simulink model "pmc"  (Simulink 7.2)
settings: Solver=ode45  StartTime=0.0  StopTime=10.0  RelTol=1e-3
libraries: cdsFilt x9, cdsMuxMatrix x9, dac x2, cdsParameters x1
settings Model: Creator=rolf  LastModifiedBy=rolf  ExtModeAutoUpdateStatusClock=off
settings OptimizationCC: InitFltsAndDblsToZero=on
settings DebuggingCC: SaveWithParameterizedLinksMsg=none  SignalResolutionControl=TryResolveAllWithWarning
settings GRTTargetCC: TargetFcnLib=ansi_tfl_tmw.mat

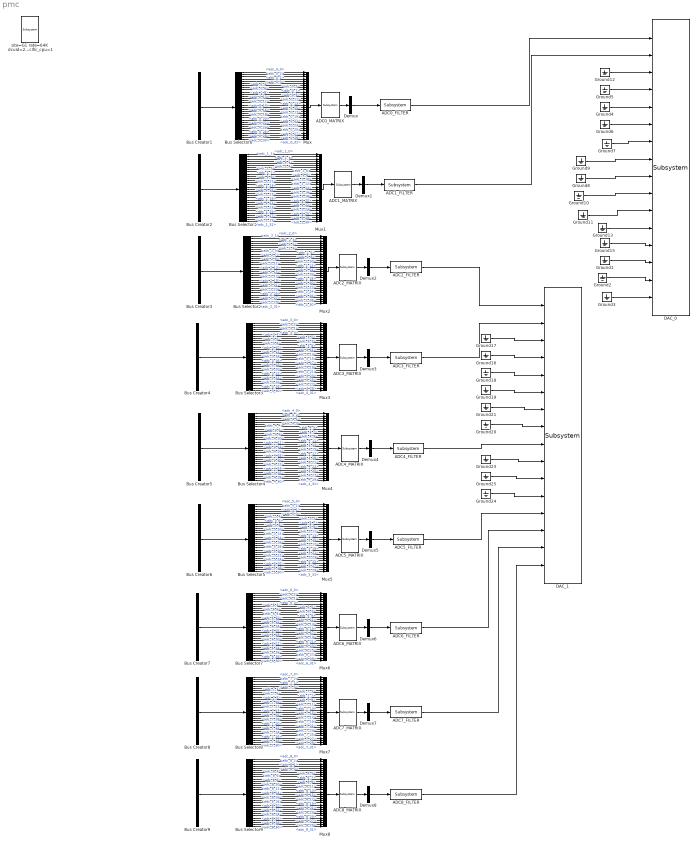
== system pmc ==
  ADC0_FILTER : cdsFilt/Subsystem  Tag=cdsFilt  Description=|  SystemSampleTime=-1
      | Purpose:                                                                                                                                                                                                                                  
      | Standard CDS IIR filter module.                                                                                                                                                                                                           
      |                                                                                                                                                                                                                                           
      | Operation:                                                                                                                                                                                                                                
      | Consists of 10 second order section IIR filters, plus a ramped gain stage. In FE code, also provides pre-defined test points and excitation channel inputs. The filter coefficients are defined in the LIGO system using the 'foton' tool.
      |                                                                                                                                                                                                                                           
      | Usage:                                                                                                                                                                                                                                    
      | Name the part with the desired filter module name.
      settings: AttributesFormatString=%<Tag>
  ADC0_MATRIX : cdsMuxMatrix/Subsystem  Tag=cdsMuxMatrix  Description=Any size matrix. Inputs and outputs must be connected using Mux and Demux parts.  SystemSampleTime=-1
      settings: AttributesFormatString=%<Tag>
  ADC1_FILTER : cdsFilt/Subsystem  Tag=cdsFilt  Description=|  SystemSampleTime=-1
      | Purpose:                                                                                                                                                                                                                                  
      | Standard CDS IIR filter module.                                                                                                                                                                                                           
      |                                                                                                                                                                                                                                           
      | Operation:                                                                                                                                                                                                                                
      | Consists of 10 second order section IIR filters, plus a ramped gain stage. In FE code, also provides pre-defined test points and excitation channel inputs. The filter coefficients are defined in the LIGO system using the 'foton' tool.
      |                                                                                                                                                                                                                                           
      | Usage:                                                                                                                                                                                                                                    
      | Name the part with the desired filter module name.
      settings: AttributesFormatString=%<Tag>
  ADC1_MATRIX : cdsMuxMatrix/Subsystem  Tag=cdsMuxMatrix  Description=Any size matrix. Inputs and outputs must be connected using Mux and Demux parts.  SystemSampleTime=-1
      settings: AttributesFormatString=%<Tag>
  ADC2_FILTER : cdsFilt/Subsystem  Tag=cdsFilt  Description=|  SystemSampleTime=-1
      | Purpose:                                                                                                                                                                                                                                  
      | Standard CDS IIR filter module.                                                                                                                                                                                                           
      |                                                                                                                                                                                                                                           
      | Operation:                                                                                                                                                                                                                                
      | Consists of 10 second order section IIR filters, plus a ramped gain stage. In FE code, also provides pre-defined test points and excitation channel inputs. The filter coefficients are defined in the LIGO system using the 'foton' tool.
      |                                                                                                                                                                                                                                           
      | Usage:                                                                                                                                                                                                                                    
      | Name the part with the desired filter module name.
      settings: AttributesFormatString=%<Tag>
  ADC2_MATRIX : cdsMuxMatrix/Subsystem  Tag=cdsMuxMatrix  Description=Any size matrix. Inputs and outputs must be connected using Mux and Demux parts.  SystemSampleTime=-1
      settings: AttributesFormatString=%<Tag>
  ADC3_FILTER : cdsFilt/Subsystem  Tag=cdsFilt  Description=|  SystemSampleTime=-1
      | Purpose:                                                                                                                                                                                                                                  
      | Standard CDS IIR filter module.                                                                                                                                                                                                           
      |                                                                                                                                                                                                                                           
      | Operation:                                                                                                                                                                                                                                
      | Consists of 10 second order section IIR filters, plus a ramped gain stage. In FE code, also provides pre-defined test points and excitation channel inputs. The filter coefficients are defined in the LIGO system using the 'foton' tool.
      |                                                                                                                                                                                                                                           
      | Usage:                                                                                                                                                                                                                                    
      | Name the part with the desired filter module name.
      settings: AttributesFormatString=%<Tag>
  ADC3_MATRIX : cdsMuxMatrix/Subsystem  Tag=cdsMuxMatrix  Description=Any size matrix. Inputs and outputs must be connected using Mux and Demux parts.  SystemSampleTime=-1
      settings: AttributesFormatString=%<Tag>
  ADC4_FILTER : cdsFilt/Subsystem  Tag=cdsFilt  Description=|  SystemSampleTime=-1
      | Purpose:                                                                                                                                                                                                                                  
      | Standard CDS IIR filter module.                                                                                                                                                                                                           
      |                                                                                                                                                                                                                                           
      | Operation:                                                                                                                                                                                                                                
      | Consists of 10 second order section IIR filters, plus a ramped gain stage. In FE code, also provides pre-defined test points and excitation channel inputs. The filter coefficients are defined in the LIGO system using the 'foton' tool.
      |                                                                                                                                                                                                                                           
      | Usage:                                                                                                                                                                                                                                    
      | Name the part with the desired filter module name.
      settings: AttributesFormatString=%<Tag>
  ADC4_MATRIX : cdsMuxMatrix/Subsystem  Tag=cdsMuxMatrix  Description=Any size matrix. Inputs and outputs must be connected using Mux and Demux parts.  SystemSampleTime=-1
      settings: AttributesFormatString=%<Tag>
  ADC5_FILTER : cdsFilt/Subsystem  Tag=cdsFilt  Description=|  SystemSampleTime=-1
      | Purpose:                                                                                                                                                                                                                                  
      | Standard CDS IIR filter module.                                                                                                                                                                                                           
      |                                                                                                                                                                                                                                           
      | Operation:                                                                                                                                                                                                                                
      | Consists of 10 second order section IIR filters, plus a ramped gain stage. In FE code, also provides pre-defined test points and excitation channel inputs. The filter coefficients are defined in the LIGO system using the 'foton' tool.
      |                                                                                                                                                                                                                                           
      | Usage:                                                                                                                                                                                                                                    
      | Name the part with the desired filter module name.
      settings: AttributesFormatString=%<Tag>
  ADC5_MATRIX : cdsMuxMatrix/Subsystem  Tag=cdsMuxMatrix  Description=Any size matrix. Inputs and outputs must be connected using Mux and Demux parts.  SystemSampleTime=-1
      settings: AttributesFormatString=%<Tag>
  ADC6_FILTER : cdsFilt/Subsystem  Tag=cdsFilt  Description=|  SystemSampleTime=-1
      | Purpose:                                                                                                                                                                                                                                  
      | Standard CDS IIR filter module.                                                                                                                                                                                                           
      |                                                                                                                                                                                                                                           
      | Operation:                                                                                                                                                                                                                                
      | Consists of 10 second order section IIR filters, plus a ramped gain stage. In FE code, also provides pre-defined test points and excitation channel inputs. The filter coefficients are defined in the LIGO system using the 'foton' tool.
      |                                                                                                                                                                                                                                           
      | Usage:                                                                                                                                                                                                                                    
      | Name the part with the desired filter module name.
      settings: AttributesFormatString=%<Tag>
  ADC6_MATRIX : cdsMuxMatrix/Subsystem  Tag=cdsMuxMatrix  Description=Any size matrix. Inputs and outputs must be connected using Mux and Demux parts.  SystemSampleTime=-1
      settings: AttributesFormatString=%<Tag>
  ADC7_FILTER : cdsFilt/Subsystem  Tag=cdsFilt  Description=|  SystemSampleTime=-1
      | Purpose:                                                                                                                                                                                                                                  
      | Standard CDS IIR filter module.                                                                                                                                                                                                           
      |                                                                                                                                                                                                                                           
      | Operation:                                                                                                                                                                                                                                
      | Consists of 10 second order section IIR filters, plus a ramped gain stage. In FE code, also provides pre-defined test points and excitation channel inputs. The filter coefficients are defined in the LIGO system using the 'foton' tool.
      |                                                                                                                                                                                                                                           
      | Usage:                                                                                                                                                                                                                                    
      | Name the part with the desired filter module name.
      settings: AttributesFormatString=%<Tag>
  ADC7_MATRIX : cdsMuxMatrix/Subsystem  Tag=cdsMuxMatrix  Description=Any size matrix. Inputs and outputs must be connected using Mux and Demux parts.  SystemSampleTime=-1
      settings: AttributesFormatString=%<Tag>
  ADC8_FILTER : cdsFilt/Subsystem  Tag=cdsFilt  Description=|  SystemSampleTime=-1
      | Purpose:                                                                                                                                                                                                                                  
      | Standard CDS IIR filter module.                                                                                                                                                                                                           
      |                                                                                                                                                                                                                                           
      | Operation:                                                                                                                                                                                                                                
      | Consists of 10 second order section IIR filters, plus a ramped gain stage. In FE code, also provides pre-defined test points and excitation channel inputs. The filter coefficients are defined in the LIGO system using the 'foton' tool.
      |                                                                                                                                                                                                                                           
      | Usage:                                                                                                                                                                                                                                    
      | Name the part with the desired filter module name.
      settings: AttributesFormatString=%<Tag>
  ADC8_MATRIX : cdsMuxMatrix/Subsystem  Tag=cdsMuxMatrix  Description=Any size matrix. Inputs and outputs must be connected using Mux and Demux parts.  SystemSampleTime=-1
      settings: AttributesFormatString=%<Tag>
  Bus Creator1 : BusCreator  Tag=adc_0  Description=|  Inputs='adc_0_0','adc_0_1','adc_0_2','adc_0_3','adc_0_4','adc_0_5','adc_0_6','adc_0_7','adc_0_8','adc_0_9','adc_0_10','adc_0_11','adc_0_12','adc_0_13','adc_0_14','adc_0_15','adc_0_16','adc_0_17','adc_0_18','adc_0_19','adc_0_20','adc_0_21','adc_0_22','adc_0_23','adc_0_24','adc_0_25','adc_0_26','adc_0_27','adc_0_28','adc_0_29','adc_0_30','adc_0_31'
      | ADC0      
      | card_num=0
      settings: AttributesFormatString=%<Description>
  Bus Creator2 : BusCreator  Description=|  Inputs='adc_1_0','adc_1_1','adc_1_2','adc_1_3','adc_1_4','adc_1_5','adc_1_6','adc_1_7','adc_1_8','adc_1_9','adc_1_10','adc_1_11','adc_1_12','adc_1_13','adc_1_14','adc_1_15','adc_1_16','adc_1_17','adc_1_18','adc_1_19','adc_1_20','adc_1_21','adc_1_22','adc_1_23','adc_1_24','adc_1_25','adc_1_26','adc_1_27','adc_1_28','adc_1_29','adc_1_30','adc_1_31'
      | ADC1      
      | card_num=1
      settings: AttributesFormatString=%<Description>
  Bus Creator3 : BusCreator  Description=|  Inputs='adc_2_0','adc_2_1','adc_2_2','adc_2_3','adc_2_4','adc_2_5','adc_2_6','adc_2_7','adc_2_8','adc_2_9','adc_2_10','adc_2_11','adc_2_12','adc_2_13','adc_2_14','adc_2_15','adc_2_16','adc_2_17','adc_2_18','adc_2_19','adc_2_20','adc_2_21','adc_2_22','adc_2_23','adc_2_24','adc_2_25','adc_2_26','adc_2_27','adc_2_28','adc_2_29','adc_2_30','adc_2_31'
      | ADC2      
      | card_num=2
      settings: AttributesFormatString=%<Description>
  Bus Creator4 : BusCreator  Description=|  Inputs='adc_3_0','adc_3_1','adc_3_2','adc_3_3','adc_3_4','adc_3_5','adc_3_6','adc_3_7','adc_3_8','adc_3_9','adc_3_10','adc_3_11','adc_3_12','adc_3_13','adc_3_14','adc_3_15','adc_3_16','adc_3_17','adc_3_18','adc_3_19','adc_3_20','adc_3_21','adc_3_22','adc_3_23','adc_3_24','adc_3_25','adc_3_26','adc_3_27','adc_3_28','adc_3_29','adc_3_30','adc_3_31'
      | ADC3      
      | card_num=3
      settings: AttributesFormatString=%<Description>
  Bus Creator5 : BusCreator  Description=|  Inputs='adc_4_0','adc_4_1','adc_4_2','adc_4_3','adc_4_4','adc_4_5','adc_4_6','adc_4_7','adc_4_8','adc_4_9','adc_4_10','adc_4_11','adc_4_12','adc_4_13','adc_4_14','adc_4_15','adc_4_16','adc_4_17','adc_4_18','adc_4_19','adc_4_20','adc_4_21','adc_4_22','adc_4_23','adc_4_24','adc_4_25','adc_4_26','adc_4_27','adc_4_28','adc_4_29','adc_4_30','adc_4_31'
      | ADC4      
      | card_num=4
      settings: AttributesFormatString=%<Description>
  Bus Creator6 : BusCreator  Description=|  Inputs='adc_5_0','adc_5_1','adc_5_2','adc_5_3','adc_5_4','adc_5_5','adc_5_6','adc_5_7','adc_5_8','adc_5_9','adc_5_10','adc_5_11','adc_5_12','adc_5_13','adc_5_14','adc_5_15','adc_5_16','adc_5_17','adc_5_18','adc_5_19','adc_5_20','adc_5_21','adc_5_22','adc_5_23','adc_5_24','adc_5_25','adc_5_26','adc_5_27','adc_5_28','adc_5_29','adc_5_30','adc_5_31'
      | ADC5      
      | card_num=5
      settings: AttributesFormatString=%<Description>
  Bus Creator7 : BusCreator  Description=|  Inputs='adc_6_0','adc_6_1','adc_6_2','adc_6_3','adc_6_4','adc_6_5','adc_6_6','adc_6_7','adc_6_8','adc_6_9','adc_6_10','adc_6_11','adc_6_12','adc_6_13','adc_6_14','adc_6_15','adc_6_16','adc_6_17','adc_6_18','adc_6_19','adc_6_20','adc_6_21','adc_6_22','adc_6_23','adc_6_24','adc_6_25','adc_6_26','adc_6_27','adc_6_28','adc_6_29','adc_6_30','adc_6_31'
      | ADC6      
      | card_num=6
      settings: AttributesFormatString=%<Description>
  Bus Creator8 : BusCreator  Description=|  Inputs='adc_7_0','adc_7_1','adc_7_2','adc_7_3','adc_7_4','adc_7_5','adc_7_6','adc_7_7','adc_7_8','adc_7_9','adc_7_10','adc_7_11','adc_7_12','adc_7_13','adc_7_14','adc_7_15','adc_7_16','adc_7_17','adc_7_18','adc_7_19','adc_7_20','adc_7_21','adc_7_22','adc_7_23','adc_7_24','adc_7_25','adc_7_26','adc_7_27','adc_7_28','adc_7_29','adc_7_30','adc_7_31'
      | ADC7      
      | card_num=7
      settings: AttributesFormatString=%<Description>
  Bus Creator9 : BusCreator  Description=|  Inputs='adc_8_0','adc_8_1','adc_8_2','adc_8_3','adc_8_4','adc_8_5','adc_8_6','adc_8_7','adc_8_8','adc_8_9','adc_8_10','adc_8_11','adc_8_12','adc_8_13','adc_8_14','adc_8_15','adc_8_16','adc_8_17','adc_8_18','adc_8_19','adc_8_20','adc_8_21','adc_8_22','adc_8_23','adc_8_24','adc_8_25','adc_8_26','adc_8_27','adc_8_28','adc_8_29','adc_8_30','adc_8_31'
      | ADC8      
      | card_num=8
      settings: AttributesFormatString=%<Description>
  Bus Selector1 : BusSelector  Description=ADC Selector  OutputSignals=adc_1_0,adc_1_1,adc_1_2,adc_1_3,adc_1_4,adc_1_5,adc_1_6,adc_1_7,adc_1_8,adc_1_9,adc_1_10,adc_1_11,adc_1_12,adc_1_13,adc_1_14,adc_1_15,adc_1_16,adc_1_17,adc_1_18,adc_1_19,adc_1_20,adc_1_21,adc_1_22,adc_1_23,adc_1_24,adc_1_25,adc_1_26,adc_1_27,adc_1_28,adc_1_29,adc_1_30,adc_1_31
      settings: AttributesFormatString=%<Description>
  Bus Selector2 : BusSelector  Description=ADC Selector  OutputSignals=adc_2_0,adc_2_1,adc_2_2,adc_2_3,adc_2_4,adc_2_5,adc_2_6,adc_2_7,adc_2_8,adc_2_9,adc_2_10,adc_2_11,adc_2_12,adc_2_13,adc_2_14,adc_2_15,adc_2_16,adc_2_17,adc_2_18,adc_2_19,adc_2_20,adc_2_21,adc_2_22,adc_2_23,adc_2_24,adc_2_25,adc_2_26,adc_2_27,adc_2_28,adc_2_29,adc_2_30,adc_2_31
      settings: AttributesFormatString=%<Description>
  Bus Selector3 : BusSelector  Description=ADC Selector  OutputSignals=adc_3_0,adc_3_1,adc_3_2,adc_3_3,adc_3_4,adc_3_5,adc_3_6,adc_3_7,adc_3_8,adc_3_9,adc_3_10,adc_3_11,adc_3_12,adc_3_13,adc_3_14,adc_3_15,adc_3_16,adc_3_17,adc_3_18,adc_3_19,adc_3_20,adc_3_21,adc_3_22,adc_3_23,adc_3_24,adc_3_25,adc_3_26,adc_3_27,adc_3_28,adc_3_29,adc_3_30,adc_3_31
      settings: AttributesFormatString=%<Description>
  Bus Selector4 : BusSelector  Description=ADC Selector  OutputSignals=adc_4_0,adc_4_1,adc_4_2,adc_4_3,adc_4_4,adc_4_5,adc_4_6,adc_4_7,adc_4_8,adc_4_9,adc_4_10,adc_4_11,adc_4_12,adc_4_13,adc_4_14,adc_4_15,adc_4_16,adc_4_17,adc_4_18,adc_4_19,adc_4_20,adc_4_21,adc_4_22,adc_4_23,adc_4_24,adc_4_25,adc_4_26,adc_4_27,adc_4_28,adc_4_29,adc_4_30,adc_4_31
      settings: AttributesFormatString=%<Description>
  Bus Selector5 : BusSelector  Description=ADC Selector  OutputSignals=adc_5_0,adc_5_1,adc_5_2,adc_5_3,adc_5_4,adc_5_5,adc_5_6,adc_5_7,adc_5_8,adc_5_9,adc_5_10,adc_5_11,adc_5_12,adc_5_13,adc_5_14,adc_5_15,adc_5_16,adc_5_17,adc_5_18,adc_5_19,adc_5_20,adc_5_21,adc_5_22,adc_5_23,adc_5_24,adc_5_25,adc_5_26,adc_5_27,adc_5_28,adc_5_29,adc_5_30,adc_5_31
      settings: AttributesFormatString=%<Description>
  Bus Selector6 : BusSelector  Description=ADC Selector  OutputSignals=adc_0_0,adc_0_1,adc_0_2,adc_0_3,adc_0_4,adc_0_5,adc_0_6,adc_0_7,adc_0_8,adc_0_9,adc_0_10,adc_0_11,adc_0_12,adc_0_13,adc_0_14,adc_0_15,adc_0_16,adc_0_17,adc_0_18,adc_0_19,adc_0_20,adc_0_21,adc_0_22,adc_0_23,adc_0_24,adc_0_25,adc_0_26,adc_0_27,adc_0_28,adc_0_29,adc_0_30,adc_0_31
      settings: AttributesFormatString=%<Description>
  Bus Selector7 : BusSelector  Description=ADC Selector  OutputSignals=adc_6_0,adc_6_1,adc_6_2,adc_6_3,adc_6_4,adc_6_5,adc_6_6,adc_6_7,adc_6_8,adc_6_9,adc_6_10,adc_6_11,adc_6_12,adc_6_13,adc_6_14,adc_6_15,adc_6_16,adc_6_17,adc_6_18,adc_6_19,adc_6_20,adc_6_21,adc_6_22,adc_6_23,adc_6_24,adc_6_25,adc_6_26,adc_6_27,adc_6_28,adc_6_29,adc_6_30,adc_6_31
      settings: AttributesFormatString=%<Description>
  Bus Selector8 : BusSelector  Description=ADC Selector  OutputSignals=adc_7_0,adc_7_1,adc_7_2,adc_7_3,adc_7_4,adc_7_5,adc_7_6,adc_7_7,adc_7_8,adc_7_9,adc_7_10,adc_7_11,adc_7_12,adc_7_13,adc_7_14,adc_7_15,adc_7_16,adc_7_17,adc_7_18,adc_7_19,adc_7_20,adc_7_21,adc_7_22,adc_7_23,adc_7_24,adc_7_25,adc_7_26,adc_7_27,adc_7_28,adc_7_29,adc_7_30,adc_7_31
      settings: AttributesFormatString=%<Description>
  Bus Selector9 : BusSelector  Description=ADC Selector  OutputSignals=adc_8_0,adc_8_1,adc_8_2,adc_8_3,adc_8_4,adc_8_5,adc_8_6,adc_8_7,adc_8_8,adc_8_9,adc_8_10,adc_8_11,adc_8_12,adc_8_13,adc_8_14,adc_8_15,adc_8_16,adc_8_17,adc_8_18,adc_8_19,adc_8_20,adc_8_21,adc_8_22,adc_8_23,adc_8_24,adc_8_25,adc_8_26,adc_8_27,adc_8_28,adc_8_29,adc_8_30,adc_8_31
      settings: AttributesFormatString=%<Description>
  DAC_0 : dac/Subsystem  Description=card_num=0  SystemSampleTime=-1
  DAC_1 : dac/Subsystem  Description=card_num=1  SystemSampleTime=-1
  Demux{,1..8} (9 alike) : Demux  Outputs=1
  Ground{1..13,15..21,23..25} (23 alike) : Ground
  Mux{,1..8} (9 alike) : Mux  Inputs=32
  site=G1 rate=64K dcuid=20 shmem_daq=1 gds_node_id=4 specific_cpu=1 : cdsParameters/Subsystem  Tag=cdsParameters  SystemSampleTime=-1
      settings: AttributesFormatString=%<Tag>
  wires:
  Ground15/1 -> DAC_0/13
  Ground1/1 -> DAC_0/14
  Ground2/1 -> DAC_0/15
  Ground3/1 -> DAC_0/16
  Bus Creator1/1 -> Bus Selector6/1
  Bus Creator2/1 -> Bus Selector1/1
  Bus Creator3/1 -> Bus Selector2/1
  Mux/1 -> ADC0_MATRIX/1
  ADC0_MATRIX/1 -> Demux/1
  Bus Selector6/1 -> Mux/1  "<adc_0_0>"
  Bus Selector6/2 -> Mux/2  "<adc_0_1>"
  Bus Selector6/3 -> Mux/3  "<adc_0_2>"
  Bus Selector6/4 -> Mux/4  "<adc_0_3>"
  Bus Selector6/5 -> Mux/5  "<adc_0_4>"
  Bus Selector6/6 -> Mux/6  "<adc_0_5>"
  Bus Selector6/7 -> Mux/7  "<adc_0_6>"
  Bus Selector6/8 -> Mux/8  "<adc_0_7>"
  Bus Selector6/9 -> Mux/9  "<adc_0_8>"
  Bus Selector6/10 -> Mux/10  "<adc_0_9>"
  Bus Selector6/11 -> Mux/11  "<adc_0_10>"
  Bus Selector6/12 -> Mux/12  "<adc_0_11>"
  Bus Selector6/13 -> Mux/13  "<adc_0_12>"
  Bus Selector6/14 -> Mux/14  "<adc_0_13>"
  Bus Selector6/15 -> Mux/15  "<adc_0_14>"
  Bus Selector6/16 -> Mux/16  "<adc_0_15>"
  Bus Selector6/17 -> Mux/17  "<adc_0_16>"
  Bus Selector6/18 -> Mux/18  "<adc_0_17>"
  Bus Selector6/19 -> Mux/19  "<adc_0_18>"
  Bus Selector6/20 -> Mux/20  "<adc_0_19>"
  Bus Selector6/21 -> Mux/21  "<adc_0_20>"
  Bus Selector6/22 -> Mux/22  "<adc_0_21>"
  Bus Selector6/23 -> Mux/23  "<adc_0_22>"
  Bus Selector6/24 -> Mux/24  "<adc_0_23>"
  Bus Selector6/25 -> Mux/25  "<adc_0_24>"
  Bus Selector6/26 -> Mux/26  "<adc_0_25>"
  Bus Selector6/27 -> Mux/27  "<adc_0_26>"
  Bus Selector6/28 -> Mux/28  "<adc_0_27>"
  Bus Selector6/29 -> Mux/29  "<adc_0_28>"
  Bus Selector6/30 -> Mux/30  "<adc_0_29>"
  Bus Selector6/31 -> Mux/31  "<adc_0_30>"
  Bus Selector6/32 -> Mux/32  "<adc_0_31>"
  Demux/1 -> ADC0_FILTER/1
  Mux1/1 -> ADC1_MATRIX/1
  ADC1_MATRIX/1 -> Demux1/1
  Bus Selector1/1 -> Mux1/1  "<adc_1_0>"
  Bus Selector1/2 -> Mux1/2  "<adc_1_1>"
  Bus Selector1/3 -> Mux1/3  "<adc_1_2>"
  Bus Selector1/4 -> Mux1/4  "<adc_1_3>"
  Bus Selector1/5 -> Mux1/5  "<adc_1_4>"
  Bus Selector1/6 -> Mux1/6  "<adc_1_5>"
  Bus Selector1/7 -> Mux1/7  "<adc_1_6>"
  Bus Selector1/8 -> Mux1/8  "<adc_1_7>"
  Bus Selector1/9 -> Mux1/9  "<adc_1_8>"
  Bus Selector1/10 -> Mux1/10  "<adc_1_9>"
  Bus Selector1/11 -> Mux1/11  "<adc_1_10>"
  Bus Selector1/12 -> Mux1/12  "<adc_1_11>"
  Bus Selector1/13 -> Mux1/13  "<adc_1_12>"
  Bus Selector1/14 -> Mux1/14  "<adc_1_13>"
  Bus Selector1/15 -> Mux1/15  "<adc_1_14>"
  Bus Selector1/16 -> Mux1/16  "<adc_1_15>"
  Bus Selector1/17 -> Mux1/17  "<adc_1_16>"
  Bus Selector1/18 -> Mux1/18  "<adc_1_17>"
  Bus Selector1/19 -> Mux1/19  "<adc_1_18>"
  Bus Selector1/20 -> Mux1/20  "<adc_1_19>"
  Bus Selector1/21 -> Mux1/21  "<adc_1_20>"
  Bus Selector1/22 -> Mux1/22  "<adc_1_21>"
  Bus Selector1/23 -> Mux1/23  "<adc_1_22>"
  Bus Selector1/24 -> Mux1/24  "<adc_1_23>"
  Bus Selector1/25 -> Mux1/25  "<adc_1_24>"
  Bus Selector1/26 -> Mux1/26  "<adc_1_25>"
  Bus Selector1/27 -> Mux1/27  "<adc_1_26>"
  Bus Selector1/28 -> Mux1/28  "<adc_1_27>"
  Bus Selector1/29 -> Mux1/29  "<adc_1_28>"
  Bus Selector1/30 -> Mux1/30  "<adc_1_29>"
  Bus Selector1/31 -> Mux1/31  "<adc_1_30>"
  Bus Selector1/32 -> Mux1/32  "<adc_1_31>"
  Mux2/1 -> ADC2_MATRIX/1
  ADC2_MATRIX/1 -> Demux2/1
  Bus Selector2/1 -> Mux2/1  "<adc_2_0>"
  Bus Selector2/2 -> Mux2/2  "<adc_2_1>"
  Bus Selector2/3 -> Mux2/3  "<adc_2_2>"
  Bus Selector2/4 -> Mux2/4  "<adc_2_3>"
  Bus Selector2/5 -> Mux2/5  "<adc_2_4>"
  Bus Selector2/6 -> Mux2/6  "<adc_2_5>"
  Bus Selector2/7 -> Mux2/7  "<adc_2_6>"
  Bus Selector2/8 -> Mux2/8  "<adc_2_7>"
  Bus Selector2/9 -> Mux2/9  "<adc_2_8>"
  Bus Selector2/10 -> Mux2/10  "<adc_2_9>"
  Bus Selector2/11 -> Mux2/11  "<adc_2_10>"
  Bus Selector2/12 -> Mux2/12  "<adc_2_11>"
  Bus Selector2/13 -> Mux2/13  "<adc_2_12>"
  Bus Selector2/14 -> Mux2/14  "<adc_2_13>"
  Bus Selector2/15 -> Mux2/15  "<adc_2_14>"
  Bus Selector2/16 -> Mux2/16  "<adc_2_15>"
  Bus Selector2/17 -> Mux2/17  "<adc_2_16>"
  Bus Selector2/18 -> Mux2/18  "<adc_2_17>"
  Bus Selector2/19 -> Mux2/19  "<adc_2_18>"
  Bus Selector2/20 -> Mux2/20  "<adc_2_19>"
  Bus Selector2/21 -> Mux2/21  "<adc_2_20>"
  Bus Selector2/22 -> Mux2/22  "<adc_2_21>"
  Bus Selector2/23 -> Mux2/23  "<adc_2_22>"
  Bus Selector2/24 -> Mux2/24  "<adc_2_23>"
  Bus Selector2/25 -> Mux2/25  "<adc_2_24>"
  Bus Selector2/26 -> Mux2/26  "<adc_2_25>"
  Bus Selector2/27 -> Mux2/27  "<adc_2_26>"
  Bus Selector2/28 -> Mux2/28  "<adc_2_27>"
  Bus Selector2/29 -> Mux2/29  "<adc_2_28>"
  Bus Selector2/30 -> Mux2/30  "<adc_2_29>"
  Bus Selector2/31 -> Mux2/31  "<adc_2_30>"
  Bus Selector2/32 -> Mux2/32  "<adc_2_31>"
  Demux2/1 -> ADC2_FILTER/1
  Demux1/1 -> ADC1_FILTER/1
  ADC0_FILTER/1 -> DAC_0/1
  ADC1_FILTER/1 -> DAC_0/2
  Ground5/1 -> DAC_0/4
  Ground4/1 -> DAC_0/5
  Ground6/1 -> DAC_0/6
  Ground7/1 -> DAC_0/7
  Ground9/1 -> DAC_0/8
  Ground8/1 -> DAC_0/9
  Ground10/1 -> DAC_0/10
  Ground11/1 -> DAC_0/11
  Ground13/1 -> DAC_0/12
  ADC2_FILTER/1 -> DAC_1/1
  Ground12/1 -> DAC_0/3
  Ground17/1 -> DAC_1/3
  Ground16/1 -> DAC_1/4
  Ground18/1 -> DAC_1/5
  Ground19/1 -> DAC_1/6
  Ground21/1 -> DAC_1/7
  Ground20/1 -> DAC_1/8
  Ground23/1 -> DAC_1/10
  Ground25/1 -> DAC_1/11
  Ground24/1 -> DAC_1/12
  Bus Creator4/1 -> Bus Selector3/1
  Mux3/1 -> ADC3_MATRIX/1
  ADC3_MATRIX/1 -> Demux3/1
  Demux3/1 -> ADC3_FILTER/1
  Bus Selector3/1 -> Mux3/1  "<adc_3_0>"
  Bus Selector3/2 -> Mux3/2  "<adc_3_1>"
  Bus Selector3/3 -> Mux3/3  "<adc_3_2>"
  Bus Selector3/4 -> Mux3/4  "<adc_3_3>"
  Bus Selector3/5 -> Mux3/5  "<adc_3_4>"
  Bus Selector3/6 -> Mux3/6  "<adc_3_5>"
  Bus Selector3/7 -> Mux3/7  "<adc_3_6>"
  Bus Selector3/8 -> Mux3/8  "<adc_3_7>"
  Bus Selector3/9 -> Mux3/9  "<adc_3_8>"
  Bus Selector3/10 -> Mux3/10  "<adc_3_9>"
  Bus Selector3/11 -> Mux3/11  "<adc_3_10>"
  Bus Selector3/12 -> Mux3/12  "<adc_3_11>"
  Bus Selector3/13 -> Mux3/13  "<adc_3_12>"
  Bus Selector3/14 -> Mux3/14  "<adc_3_13>"
  Bus Selector3/15 -> Mux3/15  "<adc_3_14>"
  Bus Selector3/16 -> Mux3/16  "<adc_3_15>"
  Bus Selector3/17 -> Mux3/17  "<adc_3_16>"
  Bus Selector3/18 -> Mux3/18  "<adc_3_17>"
  Bus Selector3/19 -> Mux3/19  "<adc_3_18>"
  Bus Selector3/20 -> Mux3/20  "<adc_3_19>"
  Bus Selector3/21 -> Mux3/21  "<adc_3_20>"
  Bus Selector3/22 -> Mux3/22  "<adc_3_21>"
  Bus Selector3/23 -> Mux3/23  "<adc_3_22>"
  Bus Selector3/24 -> Mux3/24  "<adc_3_23>"
  Bus Selector3/25 -> Mux3/25  "<adc_3_24>"
  Bus Selector3/26 -> Mux3/26  "<adc_3_25>"
  Bus Selector3/27 -> Mux3/27  "<adc_3_26>"
  Bus Selector3/28 -> Mux3/28  "<adc_3_27>"
  Bus Selector3/29 -> Mux3/29  "<adc_3_28>"
  Bus Selector3/30 -> Mux3/30  "<adc_3_29>"
  Bus Selector3/31 -> Mux3/31  "<adc_3_30>"
  Bus Selector3/32 -> Mux3/32  "<adc_3_31>"
  ADC3_FILTER/1 -> DAC_1/2
  Bus Creator5/1 -> Bus Selector4/1
  Mux4/1 -> ADC4_MATRIX/1
  ADC4_MATRIX/1 -> Demux4/1
  Demux4/1 -> ADC4_FILTER/1
  Bus Selector4/1 -> Mux4/1  "<adc_4_0>"
  Bus Selector4/2 -> Mux4/2  "<adc_4_1>"
  Bus Selector4/3 -> Mux4/3  "<adc_4_2>"
  Bus Selector4/4 -> Mux4/4  "<adc_4_3>"
  Bus Selector4/5 -> Mux4/5  "<adc_4_4>"
  Bus Selector4/6 -> Mux4/6  "<adc_4_5>"
  Bus Selector4/7 -> Mux4/7  "<adc_4_6>"
  Bus Selector4/8 -> Mux4/8  "<adc_4_7>"
  Bus Selector4/9 -> Mux4/9  "<adc_4_8>"
  Bus Selector4/10 -> Mux4/10  "<adc_4_9>"
  Bus Selector4/11 -> Mux4/11  "<adc_4_10>"
  Bus Selector4/12 -> Mux4/12  "<adc_4_11>"
  Bus Selector4/13 -> Mux4/13  "<adc_4_12>"
  Bus Selector4/14 -> Mux4/14  "<adc_4_13>"
  Bus Selector4/15 -> Mux4/15  "<adc_4_14>"
  Bus Selector4/16 -> Mux4/16  "<adc_4_15>"
  Bus Selector4/17 -> Mux4/17  "<adc_4_16>"
  Bus Selector4/18 -> Mux4/18  "<adc_4_17>"
  Bus Selector4/19 -> Mux4/19  "<adc_4_18>"
  Bus Selector4/20 -> Mux4/20  "<adc_4_19>"
  Bus Selector4/21 -> Mux4/21  "<adc_4_20>"
  Bus Selector4/22 -> Mux4/22  "<adc_4_21>"
  Bus Selector4/23 -> Mux4/23  "<adc_4_22>"
  Bus Selector4/24 -> Mux4/24  "<adc_4_23>"
  Bus Selector4/25 -> Mux4/25  "<adc_4_24>"
  Bus Selector4/26 -> Mux4/26  "<adc_4_25>"
  Bus Selector4/27 -> Mux4/27  "<adc_4_26>"
  Bus Selector4/28 -> Mux4/28  "<adc_4_27>"
  Bus Selector4/29 -> Mux4/29  "<adc_4_28>"
  Bus Selector4/30 -> Mux4/30  "<adc_4_29>"
  Bus Selector4/31 -> Mux4/31  "<adc_4_30>"
  Bus Selector4/32 -> Mux4/32  "<adc_4_31>"
  ADC4_FILTER/1 -> DAC_1/9
  Bus Creator6/1 -> Bus Selector5/1
  Mux5/1 -> ADC5_MATRIX/1
  ADC5_MATRIX/1 -> Demux5/1
  Demux5/1 -> ADC5_FILTER/1
  Bus Selector5/1 -> Mux5/1  "<adc_5_0>"
  Bus Selector5/2 -> Mux5/2  "<adc_5_1>"
  Bus Selector5/3 -> Mux5/3  "<adc_5_2>"
  Bus Selector5/4 -> Mux5/4  "<adc_5_3>"
  Bus Selector5/5 -> Mux5/5  "<adc_5_4>"
  Bus Selector5/6 -> Mux5/6  "<adc_5_5>"
  Bus Selector5/7 -> Mux5/7  "<adc_5_6>"
  Bus Selector5/8 -> Mux5/8  "<adc_5_7>"
  Bus Selector5/9 -> Mux5/9  "<adc_5_8>"
  Bus Selector5/10 -> Mux5/10  "<adc_5_9>"
  Bus Selector5/11 -> Mux5/11  "<adc_5_10>"
  Bus Selector5/12 -> Mux5/12  "<adc_5_11>"
  Bus Selector5/13 -> Mux5/13  "<adc_5_12>"
  Bus Selector5/14 -> Mux5/14  "<adc_5_13>"
  Bus Selector5/15 -> Mux5/15  "<adc_5_14>"
  Bus Selector5/16 -> Mux5/16  "<adc_5_15>"
  Bus Selector5/17 -> Mux5/17  "<adc_5_16>"
  Bus Selector5/18 -> Mux5/18  "<adc_5_17>"
  Bus Selector5/19 -> Mux5/19  "<adc_5_18>"
  Bus Selector5/20 -> Mux5/20  "<adc_5_19>"
  Bus Selector5/21 -> Mux5/21  "<adc_5_20>"
  Bus Selector5/22 -> Mux5/22  "<adc_5_21>"
  Bus Selector5/23 -> Mux5/23  "<adc_5_22>"
  Bus Selector5/24 -> Mux5/24  "<adc_5_23>"
  Bus Selector5/25 -> Mux5/25  "<adc_5_24>"
  Bus Selector5/26 -> Mux5/26  "<adc_5_25>"
  Bus Selector5/27 -> Mux5/27  "<adc_5_26>"
  Bus Selector5/28 -> Mux5/28  "<adc_5_27>"
  Bus Selector5/29 -> Mux5/29  "<adc_5_28>"
  Bus Selector5/30 -> Mux5/30  "<adc_5_29>"
  Bus Selector5/31 -> Mux5/31  "<adc_5_30>"
  Bus Selector5/32 -> Mux5/32  "<adc_5_31>"
  ADC5_FILTER/1 -> DAC_1/13
  Bus Creator7/1 -> Bus Selector7/1
  Mux6/1 -> ADC6_MATRIX/1
  ADC6_MATRIX/1 -> Demux6/1
  Demux6/1 -> ADC6_FILTER/1
  Bus Selector7/1 -> Mux6/1  "<adc_6_0>"
  Bus Selector7/2 -> Mux6/2  "<adc_6_1>"
  Bus Selector7/3 -> Mux6/3  "<adc_6_2>"
  Bus Selector7/4 -> Mux6/4  "<adc_6_3>"
  Bus Selector7/5 -> Mux6/5  "<adc_6_4>"
  Bus Selector7/6 -> Mux6/6  "<adc_6_5>"
  Bus Selector7/7 -> Mux6/7  "<adc_6_6>"
  Bus Selector7/8 -> Mux6/8  "<adc_6_7>"
  Bus Selector7/9 -> Mux6/9  "<adc_6_8>"
  Bus Selector7/10 -> Mux6/10  "<adc_6_9>"
  Bus Selector7/11 -> Mux6/11  "<adc_6_10>"
  Bus Selector7/12 -> Mux6/12  "<adc_6_11>"
  Bus Selector7/13 -> Mux6/13  "<adc_6_12>"
  Bus Selector7/14 -> Mux6/14  "<adc_6_13>"
  Bus Selector7/15 -> Mux6/15  "<adc_6_14>"
  Bus Selector7/16 -> Mux6/16  "<adc_6_15>"
  Bus Selector7/17 -> Mux6/17  "<adc_6_16>"
  Bus Selector7/18 -> Mux6/18  "<adc_6_17>"
  Bus Selector7/19 -> Mux6/19  "<adc_6_18>"
  Bus Selector7/20 -> Mux6/20  "<adc_6_19>"
  Bus Selector7/21 -> Mux6/21  "<adc_6_20>"
  Bus Selector7/22 -> Mux6/22  "<adc_6_21>"
  Bus Selector7/23 -> Mux6/23  "<adc_6_22>"
  Bus Selector7/24 -> Mux6/24  "<adc_6_23>"
  Bus Selector7/25 -> Mux6/25  "<adc_6_24>"
  Bus Selector7/26 -> Mux6/26  "<adc_6_25>"
  Bus Selector7/27 -> Mux6/27  "<adc_6_26>"
  Bus Selector7/28 -> Mux6/28  "<adc_6_27>"
  Bus Selector7/29 -> Mux6/29  "<adc_6_28>"
  Bus Selector7/30 -> Mux6/30  "<adc_6_29>"
  Bus Selector7/31 -> Mux6/31  "<adc_6_30>"
  Bus Selector7/32 -> Mux6/32  "<adc_6_31>"
  ADC6_FILTER/1 -> DAC_1/14
  Bus Creator8/1 -> Bus Selector8/1
  Mux7/1 -> ADC7_MATRIX/1
  ADC7_MATRIX/1 -> Demux7/1
  Demux7/1 -> ADC7_FILTER/1
  Bus Selector8/1 -> Mux7/1  "<adc_7_0>"
  Bus Selector8/2 -> Mux7/2  "<adc_7_1>"
  Bus Selector8/3 -> Mux7/3  "<adc_7_2>"
  Bus Selector8/4 -> Mux7/4  "<adc_7_3>"
  Bus Selector8/5 -> Mux7/5  "<adc_7_4>"
  Bus Selector8/6 -> Mux7/6  "<adc_7_5>"
  Bus Selector8/7 -> Mux7/7  "<adc_7_6>"
  Bus Selector8/8 -> Mux7/8  "<adc_7_7>"
  Bus Selector8/9 -> Mux7/9  "<adc_7_8>"
  Bus Selector8/10 -> Mux7/10  "<adc_7_9>"
  Bus Selector8/11 -> Mux7/11  "<adc_7_10>"
  Bus Selector8/12 -> Mux7/12  "<adc_7_11>"
  Bus Selector8/13 -> Mux7/13  "<adc_7_12>"
  Bus Selector8/14 -> Mux7/14  "<adc_7_13>"
  Bus Selector8/15 -> Mux7/15  "<adc_7_14>"
  Bus Selector8/16 -> Mux7/16  "<adc_7_15>"
  Bus Selector8/17 -> Mux7/17  "<adc_7_16>"
  Bus Selector8/18 -> Mux7/18  "<adc_7_17>"
  Bus Selector8/19 -> Mux7/19  "<adc_7_18>"
  Bus Selector8/20 -> Mux7/20  "<adc_7_19>"
  Bus Selector8/21 -> Mux7/21  "<adc_7_20>"
  Bus Selector8/22 -> Mux7/22  "<adc_7_21>"
  Bus Selector8/23 -> Mux7/23  "<adc_7_22>"
  Bus Selector8/24 -> Mux7/24  "<adc_7_23>"
  Bus Selector8/25 -> Mux7/25  "<adc_7_24>"
  Bus Selector8/26 -> Mux7/26  "<adc_7_25>"
  Bus Selector8/27 -> Mux7/27  "<adc_7_26>"
  Bus Selector8/28 -> Mux7/28  "<adc_7_27>"
  Bus Selector8/29 -> Mux7/29  "<adc_7_28>"
  Bus Selector8/30 -> Mux7/30  "<adc_7_29>"
  Bus Selector8/31 -> Mux7/31  "<adc_7_30>"
  Bus Selector8/32 -> Mux7/32  "<adc_7_31>"
  ADC7_FILTER/1 -> DAC_1/15
  Bus Creator9/1 -> Bus Selector9/1
  Mux8/1 -> ADC8_MATRIX/1
  ADC8_MATRIX/1 -> Demux8/1
  Demux8/1 -> ADC8_FILTER/1
  Bus Selector9/1 -> Mux8/1  "<adc_8_0>"
  Bus Selector9/2 -> Mux8/2  "<adc_8_1>"
  Bus Selector9/3 -> Mux8/3  "<adc_8_2>"
  Bus Selector9/4 -> Mux8/4  "<adc_8_3>"
  Bus Selector9/5 -> Mux8/5  "<adc_8_4>"
  Bus Selector9/6 -> Mux8/6  "<adc_8_5>"
  Bus Selector9/7 -> Mux8/7  "<adc_8_6>"
  Bus Selector9/8 -> Mux8/8  "<adc_8_7>"
  Bus Selector9/9 -> Mux8/9  "<adc_8_8>"
  Bus Selector9/10 -> Mux8/10  "<adc_8_9>"
  Bus Selector9/11 -> Mux8/11  "<adc_8_10>"
  Bus Selector9/12 -> Mux8/12  "<adc_8_11>"
  Bus Selector9/13 -> Mux8/13  "<adc_8_12>"
  Bus Selector9/14 -> Mux8/14  "<adc_8_13>"
  Bus Selector9/15 -> Mux8/15  "<adc_8_14>"
  Bus Selector9/16 -> Mux8/16  "<adc_8_15>"
  Bus Selector9/17 -> Mux8/17  "<adc_8_16>"
  Bus Selector9/18 -> Mux8/18  "<adc_8_17>"
  Bus Selector9/19 -> Mux8/19  "<adc_8_18>"
  Bus Selector9/20 -> Mux8/20  "<adc_8_19>"
  Bus Selector9/21 -> Mux8/21  "<adc_8_20>"
  Bus Selector9/22 -> Mux8/22  "<adc_8_21>"
  Bus Selector9/23 -> Mux8/23  "<adc_8_22>"
  Bus Selector9/24 -> Mux8/24  "<adc_8_23>"
  Bus Selector9/25 -> Mux8/25  "<adc_8_24>"
  Bus Selector9/26 -> Mux8/26  "<adc_8_25>"
  Bus Selector9/27 -> Mux8/27  "<adc_8_26>"
  Bus Selector9/28 -> Mux8/28  "<adc_8_27>"
  Bus Selector9/29 -> Mux8/29  "<adc_8_28>"
  Bus Selector9/30 -> Mux8/30  "<adc_8_29>"
  Bus Selector9/31 -> Mux8/31  "<adc_8_30>"
  Bus Selector9/32 -> Mux8/32  "<adc_8_31>"
  ADC8_FILTER/1 -> DAC_1/16
